simulink model "zad2_system"  (R2023b)
settings: Solver=VariableStepAuto  StartTime=0.0  StopTime=100  RelTol=1e-3
values from neighbouring files (symbols this model uses):
  a = 0.01    [zad2.m]
  alfa = 0.5    [zad2.m]
  beta = 1    [zad2.m]
  K = 0.5    [zad2.m]
  k = 0.5    [zad2.m]
  m = 1    [zad2.m]
  w0 = 0    [zad2.m]
  x0 = 0.5    [zad2.m]
  x0_poch = 0    [zad2.m]
settings Model: Creator=student  LastModifiedBy=roman

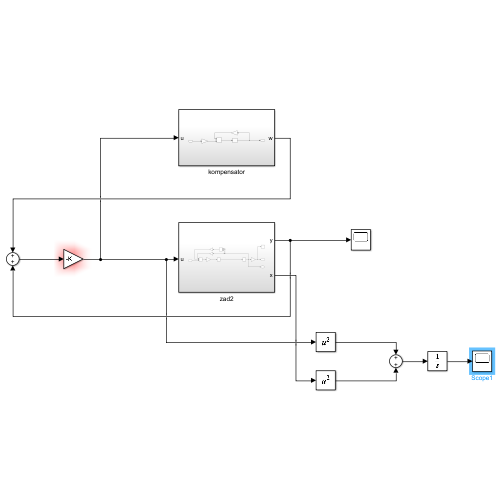
[thumbnail: Simulink's stored preview of the top-level diagram]
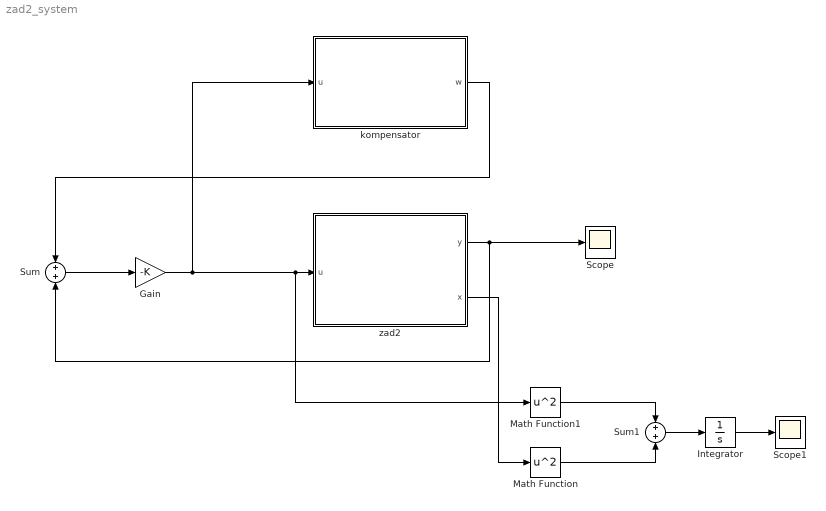
== system zad2_system ==
  Gain : Gain  Gain=-K
  Integrator : Integrator
  Math Function : Math  Operator=square
  Math Function1 : Math  Operator=square
  Scope : Scope
  Scope1 : Scope
  Sum : Sum
  Sum1 : Sum
  kompensator : Subsystem
  zad2 : Subsystem
  wires:
  Sum/1 -> Gain/1
  zad2/1(y) -> Sum/2, Scope/1
  kompensator/1(w) -> Sum/1
  Gain/1 -> kompensator/1(u), Math Function1/1, zad2/1(u)
  Math Function1/1 -> Sum1/1
  Math Function/1 -> Sum1/2
  zad2/2(x) -> Math Function/1
  Sum1/1 -> Integrator/1
  Integrator/1 -> Scope1/1

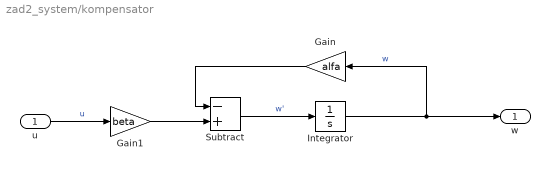
== system zad2_system/kompensator ==
  u : Inport
  Gain : Gain  Gain=alfa
  Gain1 : Gain  Gain=beta
  Integrator : Integrator  InitialCondition=w0
  Subtract : Sum  Inputs=-+
  w : Outport
  wires:
  Subtract/1 -> Integrator/1  "w'"
  u/1 -> Gain1/1  "u"
  Integrator/1 -> w/1, Gain/1  "w"
  Gain/1 -> Subtract/1
  Gain1/1 -> Subtract/2

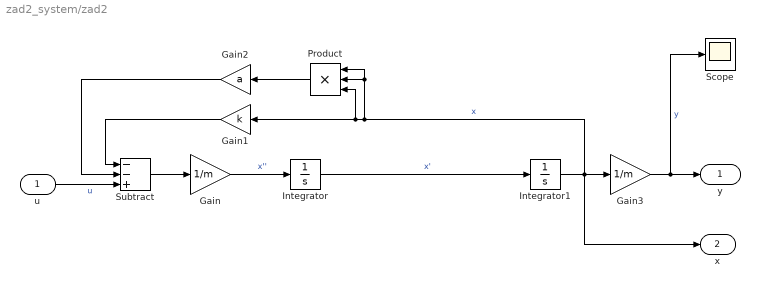
== system zad2_system/zad2 ==
  u : Inport
  Gain : Gain  Gain=1/m
  Gain1 : Gain  Gain=k
  Gain2 : Gain  Gain=a
  Gain3 : Gain  Gain=1/m
  Integrator : Integrator  InitialCondition=x0_poch
  Integrator1 : Integrator  InitialCondition=x0
  Product : Product  Inputs=3
  Scope : Scope
  Subtract : Sum  Inputs=--+
  y : Outport
  x : Outport  Port=2
  wires:
  u/1 -> Subtract/3  "u"
  Gain3/1 -> Scope/1, y/1  "y"
  Product/1 -> Gain2/1
  Gain/1 -> Integrator/1  "x''"
  Gain1/1 -> Subtract/1
  Gain2/1 -> Subtract/2
  Integrator1/1 -> x/1, Gain3/1, Gain1/1, Product/3, Product/1, Product/2  "x"
  Integrator/1 -> Integrator1/1  "x'"
  Subtract/1 -> Gain/1
